simulink model "Control_schemes"  (R2022b)
settings: Solver=VariableStepAuto  StartTime=0.0  StopTime=50  RelTol=1e-3
undefined symbols (not defined in the file or in its folder): K_lqr, sigbuilder_block
libraries: simulink_extras x7, cstblocks x5
settings Model: Creator=AleFire  LastModifiedBy=alefi

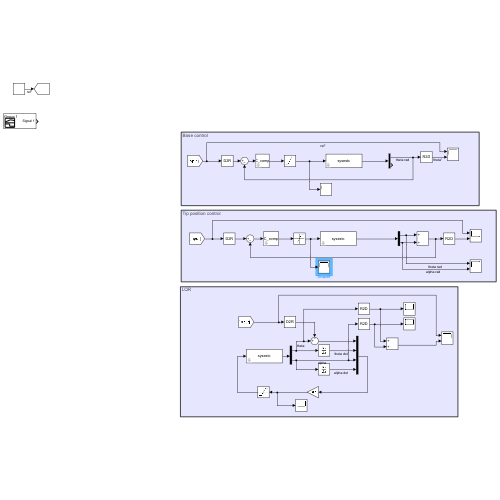
[thumbnail: Simulink's stored preview of the top-level diagram]
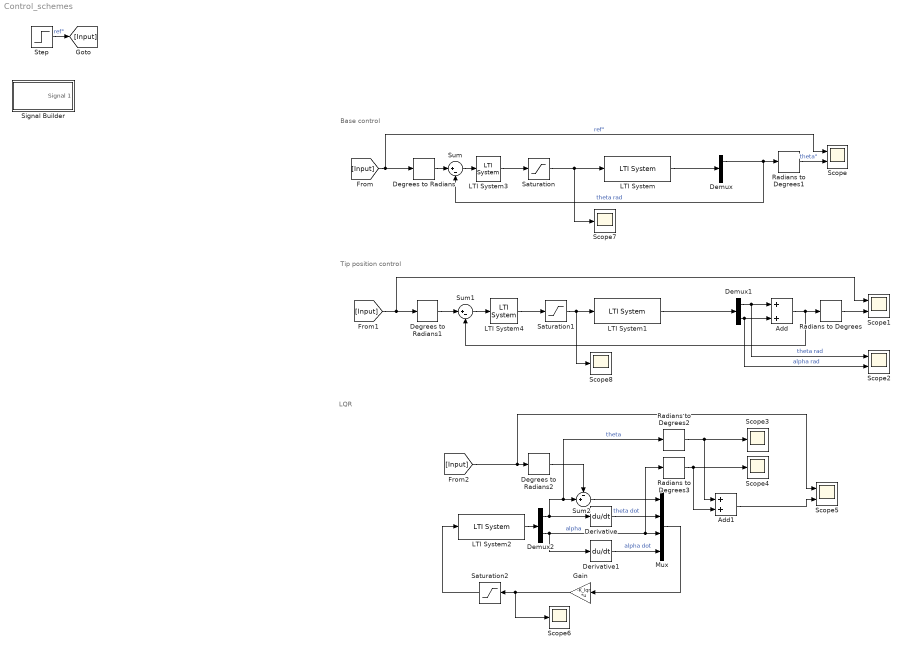
== system Control_schemes ==
  note: LQR
  note: Tip position control
  note: Base control
  Add : Sum
  Add1 : Sum
  Degrees to Radians : simulink_extras/Transformations/Degrees to Radians
  Degrees to Radians1 : simulink_extras/Transformations/Degrees to Radians
  Degrees to Radians2 : simulink_extras/Transformations/Degrees to Radians
  Demux : Demux  Outputs=2
  Demux1 : Demux  Outputs=2
  Demux2 : Demux  Outputs=2
  Derivative : Derivative
  Derivative1 : Derivative
  Gain : Gain  Gain=-K_lqr  Multiplication=Matrix(K*u)
  LTI System : cstblocks/LTI System  sys=sysestc  IC=[]
  LTI System1 : cstblocks/LTI System  sys=sysestc  IC=[]
  LTI System2 : cstblocks/LTI System  sys=sysestc  IC=[]
  LTI System3 : cstblocks/LTI System  sys=C_comp  IC=[]
  LTI System4 : cstblocks/LTI System  sys=C_comp  IC=[]
  Mux : Mux
  Radians to Degrees{,1..3} (4 alike) : simulink_extras/Transformations/Radians to Degrees
  Saturation : Saturate  UpperLimit=4.5  LowerLimit=-4.5
  Saturation1 : Saturate  UpperLimit=4.5  LowerLimit=-4.5
  Saturation2 : Saturate  UpperLimit=4.5  LowerLimit=-4.5
  Scope{,1..2,5} (4 alike) : Scope  NumInputPorts=2
  Scope{3..4,6..8} (5 alike) : Scope
  Signal Builder : Subsystem  Tag=STV Subsys  LoadFcn=sigbuilder_block('load');  StartFcn=sigbuilder_block('start');  StopFcn=sigbuilder_block('stop');  ClipboardFcn=sigbuilder_block('clipboard');  mask(Sigbuilder block){tuvar=[0:10]}
      mask help: Simulink:masks:SigbuilderBlock_MD
      mask init:
      | if ~strcmp(get_param(bdroot(gcbh),'SimulationStatus'),'stopped') tuvar = sigbuilder_block('maskInit'); end
      settings: CopyFcn=sigbuilder_block('copy');  DeleteFcn=sigbuilder_block('delete');  ModelCloseFcn=sigbuilder_block('modelClose');  PreSaveFcn=sigbuilder_block('preSave');  PauseFcn=sigbuilder_block('pause');  ContinueFcn=sigbuilder_block('continue');  NameChangeFcn=sigbuilder_block('namechange');  OpenFcn=sigbuilder_block('open',[437.6 199.2 550.4 400 ]);  CloseFcn=sigbuilder_block('close');
      mask Display: plot(0, 0, 100, 100,[2, 2, 32, 32, 2], [68, 8, 8, 68, 68],[32, 2], [38, 38], [32, 19, 2],[53, 60, 44], [32, 17, 17, 2],[16, 16, 31, 31]);txt = getActiveGroup(gcbh);text(2, 100, txt,'verticalAlignment', 'top');
  Step : Step  After=20  SampleTime=0
  Sum : Sum  Inputs=|+-
  Sum1 : Sum  Inputs=|+-
  Sum2 : Sum  Inputs=-+|
  wires:
  [Input] -> Degrees to Radians/1, Scope/1  "ref°"
  Degrees to Radians/1 -> Sum/1
  Demux/1 -> Radians to Degrees1/1, Sum/2  "theta rad"
  LTI System/1 -> Demux/1
  Radians to Degrees1/1 -> Scope/2  "theta°"
  Radians to Degrees/1 -> Scope1/2
  Add/1 -> Radians to Degrees/1, Sum1/2
  LTI System1/1 -> Demux1/1
  Degrees to Radians1/1 -> Sum1/1
  [Input] -> Degrees to Radians1/1, Scope1/1
  Demux1/1 -> Scope2/1, Add/1  "theta rad"
  Demux1/2 -> Scope2/2, Add/2  "alpha rad"
  Degrees to Radians2/1 -> Sum2/1
  LTI System2/1 -> Demux2/1
  Demux2/1 -> Radians to Degrees2/1, Sum2/2, Derivative/1  "theta"
  Derivative/1 -> Mux/2  "theta dot"
  Mux/1 -> Gain/1
  Demux2/2 -> Derivative1/1, Radians to Degrees3/1, Mux/3  "alpha"
  Derivative1/1 -> Mux/4  "alpha dot"
  Gain/1 -> Saturation2/1, Scope6/1
  Sum2/1 -> Mux/1
  Radians to Degrees2/1 -> Add1/1, Scope3/1
  Radians to Degrees3/1 -> Add1/2, Scope4/1
  Add1/1 -> Scope5/2
  [Input] -> Scope5/1, Degrees to Radians2/1
  Sum1/1 -> LTI System4/1
  Sum/1 -> LTI System3/1
  Step/1 -> [Input]  "ref°"
  LTI System3/1 -> Saturation/1
  Saturation/1 -> Scope7/1, LTI System/1
  Saturation1/1 -> Scope8/1, LTI System1/1
  LTI System4/1 -> Saturation1/1
  Saturation2/1 -> LTI System2/1

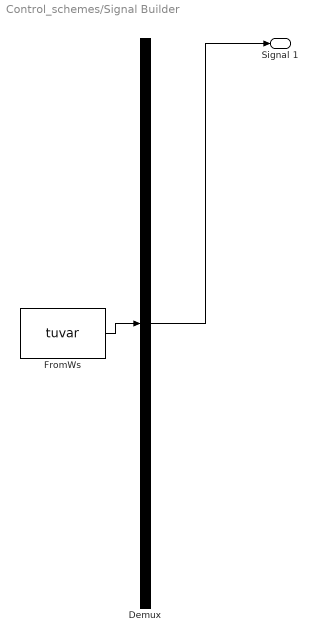
== system Control_schemes/Signal Builder ==
  Demux : Demux  Tag=STV Demux  Outputs=1
      settings: DisplayOption=none
  FromWs : FromWorkspace  Tag=STV FromWs  VariableName=tuvar
      SigBuilderData=|
      | common.afterFinalStr = 'Extrapolate'
      | common.sampleTime = 0
      | dataSet.timeRange = [0 10]
      | dataSet.name = 'Group 1'
      | sbobj.Groups.Name = 'Group 1'
      | sbobj.Groups.Signals.Name = 'Signal 1'
      | sbobj.Groups.Signals.XData = [0 0.94 2 2 2.82 4 4 6 6 7.6 10]
      | sbobj.Groups.Signals.YData = [0 1.015 1.01 -0.285 0.83 0.125 0.665 0.785 -0.24 -0.325 0]
  Signal 1 : Outport  Tag=STV Outport
  wires:
  Demux/1 -> Signal 1/1
  FromWs/1 -> Demux/1
